simulink model "ADCS_sim"  (R2021b)
settings: Solver=VariableStepAuto  StartTime=0.0  StopTime=tf  RelTol=1e-3
values from neighbouring files (symbols this model uses):
  q_i = flip(quat)    [Jeri_Attitude_Prop.m]    (also in Nova_Attitude_Prop2.m = flip(q_i))
  w_i = [P;Q;R]    [Jeri_Attitude_Prop.m]    (also in Nova_Attitude_Prop2.m = [p;q;r])
undefined symbols (not defined in the file or in its folder): Params, qc, wc
libraries: sharedutil x1
settings Model: Creator=orena  LastModifiedBy=Tom
settings SolverCC: AlgebraicLoopSolver=TrustRegion
settings DebuggingCC: SFMachineParentedDataDiag=warning

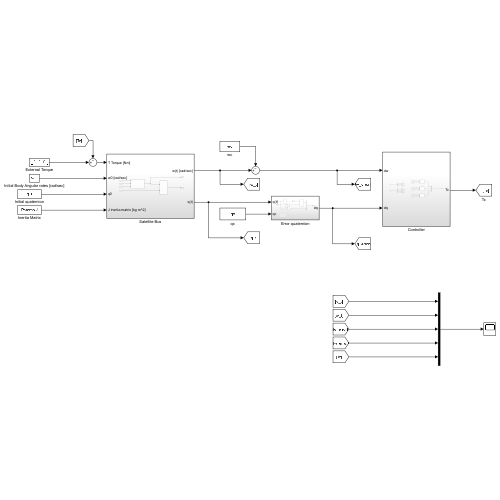
[thumbnail: Simulink's stored preview of the top-level diagram]
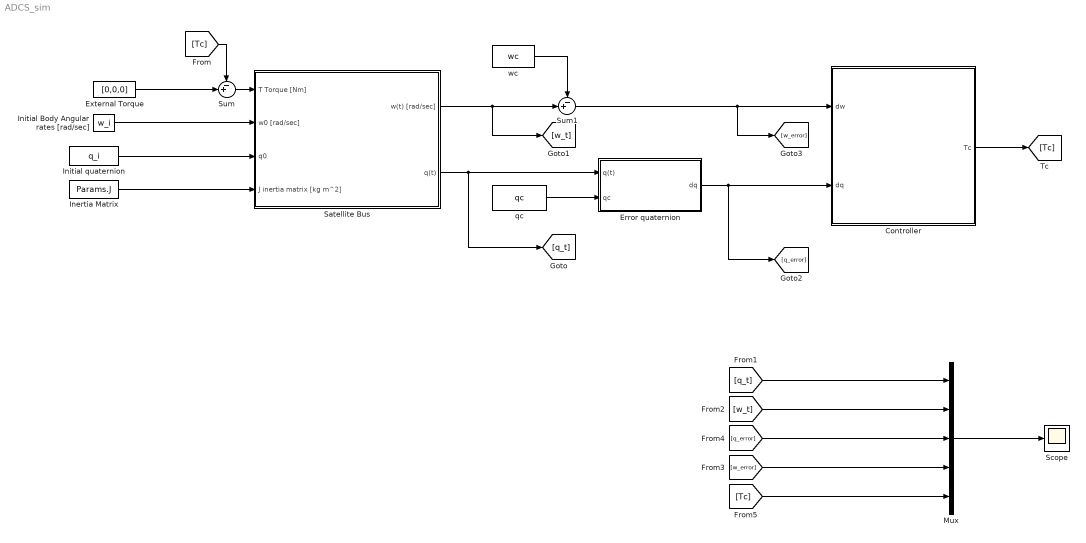
== system ADCS_sim ==
  Controller : Subsystem
  Error quaternion : Subsystem
  External Torque : Constant  Value=[0,0,0]
  Inertia Matrix : Constant  Value=Params.J
  Initial Body Angular rates [rad/sec] : Constant  Value=w_i
  Initial quaternion : Constant  Value=q_i
  Mux : Mux  Inputs=5
  Satellite Bus : Subsystem
  Scope : Scope
  Sum : Sum  Inputs=-+|
  Sum1 : Sum  Inputs=-+|
  qc : Constant  Value=qc
  wc : Constant  Value=wc
  wires:
  External Torque/1 -> Sum/2
  Controller/1(Tc) -> [Tc]
  [Tc] -> Sum/1
  wc/1 -> Sum1/1
  Sum/1 -> Satellite Bus/1(T Torque [Nm])
  Initial Body Angular rates [rad/sec]/1 -> Satellite Bus/2(w0 [rad/sec])
  Inertia Matrix/1 -> Satellite Bus/4(J inertia matrix [kg m^2])
  qc/1 -> Error quaternion/2(qc)
  Satellite Bus/2(q(t)) -> [q_t], Error quaternion/1(q(t))
  Error quaternion/1(dq) -> Controller/2(dq), [q_error]
  Satellite Bus/1(w(t) [rad/sec]) -> [w_t], Sum1/2
  Sum1/1 -> [w_error], Controller/1(dw)
  Initial quaternion/1 -> Satellite Bus/3(q0)
  [Tc] -> Mux/5
  [q_t] -> Mux/1
  [w_t] -> Mux/2
  [q_error] -> Mux/3
  [w_error] -> Mux/4
  Mux/1 -> Scope/1

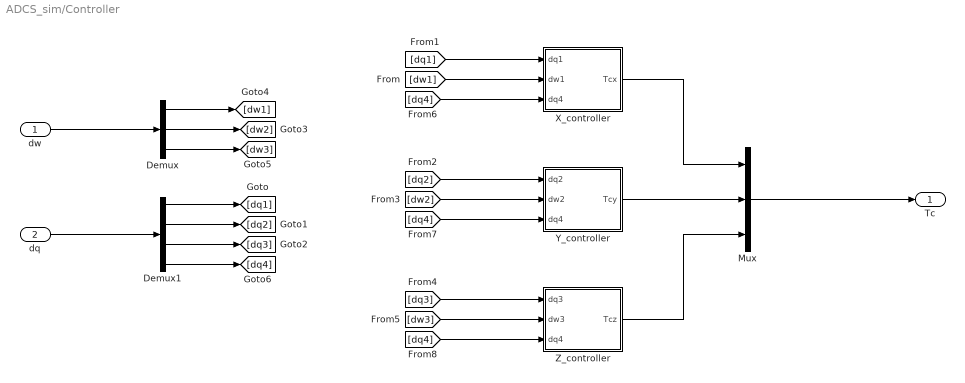
== system ADCS_sim/Controller ==
  dw : Inport
  dq : Inport  Port=2
  Demux : Demux  Outputs=3
  Demux1 : Demux
  Mux : Mux  Inputs=3
  X_controller : Subsystem
  Y_controller : Subsystem
  Z_controller : Subsystem
  Tc : Outport
  wires:
  Demux/1 -> [dw1]
  [dw2] -> Y_controller/2(dw2)
  [dq1] -> X_controller/1(dq1)
  [dq3] -> Z_controller/1(dq3)
  Demux/2 -> [dw2]
  Demux/3 -> [dw3]
  [dw3] -> Z_controller/2(dw3)
  Demux1/3 -> [dq3]
  Demux1/1 -> [dq1]
  Demux1/2 -> [dq2]
  [dq2] -> Y_controller/1(dq2)
  dw/1 -> Demux/1
  [dw1] -> X_controller/2(dw1)
  Y_controller/1(Tcy) -> Mux/2
  X_controller/1(Tcx) -> Mux/1
  Z_controller/1(Tcz) -> Mux/3
  Mux/1 -> Tc/1
  dq/1 -> Demux1/1
  Demux1/4 -> [dq4]
  [dq4] -> X_controller/3(dq4)
  [dq4] -> Y_controller/3(dq4)
  [dq4] -> Z_controller/3(dq4)

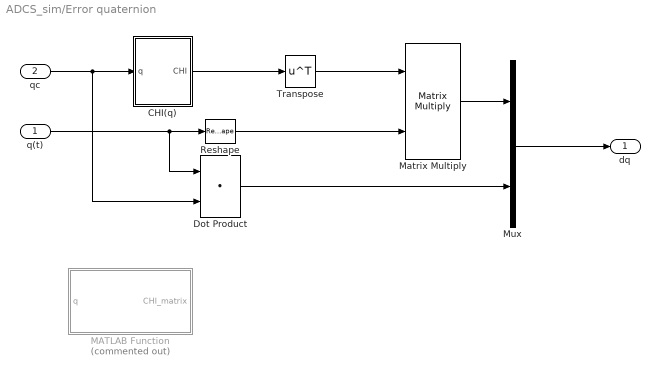
== system ADCS_sim/Error quaternion ==
  q(t) : Inport
  qc : Inport  Port=2
  CHI(q) : Subsystem
  Dot Product : DotProduct  InputSameDT=on  OutDataTypeStr=Inherit: Inherit via internal rule
  MATLAB Function : MATLAB Function  Commented=on  TreatAsAtomicUnit=on
  Matrix Multiply : Product  Multiplication=Matrix(*)
  Mux : Mux  Inputs=2
  Reshape : Reshape  OutputDimensionality=Column vector (2-D)
  Transpose : Math  Operator=transpose  SaturateOnIntegerOverflow=on
  dq : Outport
  wires:
  q(t)/1 -> Dot Product/1, Reshape/1
  Reshape/1 -> Matrix Multiply/2
  CHI(q)/1(CHI) -> Transpose/1
  qc/1 -> Dot Product/2, CHI(q)/1(q)
  Transpose/1 -> Matrix Multiply/1
  Matrix Multiply/1 -> Mux/1
  Mux/1 -> dq/1
  Dot Product/1 -> Mux/2

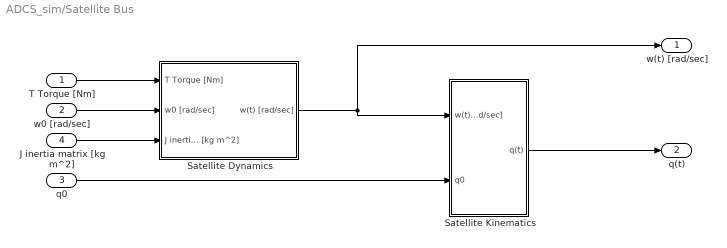
== system ADCS_sim/Satellite Bus ==
  T Torque [Nm] : Inport
  w0 [rad/sec] : Inport  Port=2
  q0 : Inport  Port=3
  J inertia matrix [kg m^2] : Inport  Port=4
  Satellite Dynamics : Subsystem
  Satellite Kinematics : Subsystem
  w(t) [rad/sec] : Outport
  q(t) : Outport  Port=2
  wires:
  q0/1 -> Satellite Kinematics/2(q0)
  Satellite Kinematics/1(q(t)) -> q(t)/1
  J inertia matrix [kg m^2]/1 -> Satellite Dynamics/3(J inertia matrix [kg m^2])
  w0 [rad/sec]/1 -> Satellite Dynamics/2(w0 [rad/sec])
  Satellite Dynamics/1(w(t) [rad/sec]) -> Satellite Kinematics/1(w(t) [rad/sec]), w(t) [rad/sec]/1
  T Torque [Nm]/1 -> Satellite Dynamics/1(T Torque [Nm])

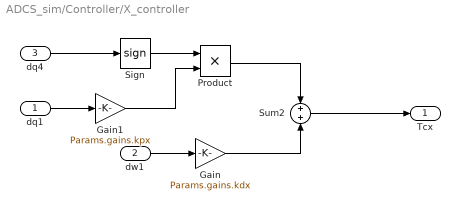
== system ADCS_sim/Controller/X_controller ==
  dq1 : Inport
  dw1 : Inport  Port=2
  dq4 : Inport  Port=3
  Gain : Gain  Gain=Params.gains.kdx
  Gain1 : Gain  Gain=Params.gains.kpx
  Product : Product
  Sign : Signum
  Sum2 : Sum  Inputs=+|+
  Tcx : Outport
  wires:
  Sum2/1 -> Tcx/1
  dq1/1 -> Gain1/1
  dw1/1 -> Gain/1
  Gain/1 -> Sum2/2
  dq4/1 -> Sign/1
  Sign/1 -> Product/1
  Gain1/1 -> Product/2
  Product/1 -> Sum2/1

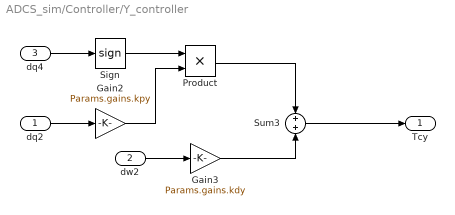
== system ADCS_sim/Controller/Y_controller ==
  dq2 : Inport
  dw2 : Inport  Port=2
  dq4 : Inport  Port=3
  Gain2 : Gain  Gain=Params.gains.kpy
  Gain3 : Gain  Gain=Params.gains.kdy
  Product : Product
  Sign : Signum
  Sum3 : Sum  Inputs=+|+
  Tcy : Outport
  wires:
  dq2/1 -> Gain2/1
  Gain3/1 -> Sum3/2
  Sum3/1 -> Tcy/1
  dw2/1 -> Gain3/1
  dq4/1 -> Sign/1
  Sign/1 -> Product/1
  Gain2/1 -> Product/2
  Product/1 -> Sum3/1

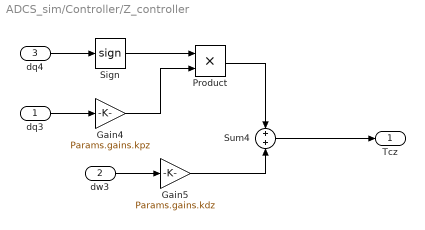
== system ADCS_sim/Controller/Z_controller ==
  dq3 : Inport
  dw3 : Inport  Port=2
  dq4 : Inport  Port=3
  Gain4 : Gain  Gain=Params.gains.kpz
  Gain5 : Gain  Gain=Params.gains.kdz
  Product : Product
  Sign : Signum
  Sum4 : Sum  Inputs=+|+
  Tcz : Outport
  wires:
  Sum4/1 -> Tcz/1
  dw3/1 -> Gain5/1
  Gain5/1 -> Sum4/2
  dq3/1 -> Gain4/1
  dq4/1 -> Sign/1
  Sign/1 -> Product/1
  Gain4/1 -> Product/2
  Product/1 -> Sum4/1

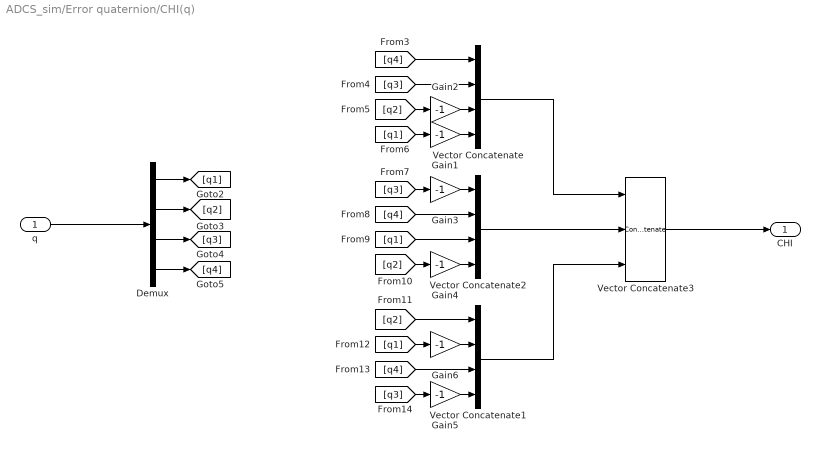
== system ADCS_sim/Error quaternion/CHI(q) ==
  q : Inport
  Demux : Demux
  Gain{1..6} (6 alike) : Gain  Gain=-1
  Vector Concatenate : Concatenate  NumInputs=4
  Vector Concatenate1 : Concatenate  NumInputs=4
  Vector Concatenate2 : Concatenate  NumInputs=4
  Vector Concatenate3 : Concatenate  NumInputs=3  Mode=Multidimensional array  ConcatenateDimension=2
  CHI : Outport
  wires:
  [q1] -> Vector Concatenate2/3
  [q3] -> Gain5/1
  Vector Concatenate3/1 -> CHI/1
  Vector Concatenate/1 -> Vector Concatenate3/1
  Vector Concatenate2/1 -> Vector Concatenate3/2
  q/1 -> Demux/1
  [q3] -> Gain3/1
  Gain3/1 -> Vector Concatenate2/1
  [q3] -> Vector Concatenate/2
  [q4] -> Vector Concatenate1/3
  [q1] -> Gain1/1
  Demux/2 -> [q2]
  Gain1/1 -> Vector Concatenate/4
  Demux/3 -> [q3]
  [q4] -> Vector Concatenate/1
  [q4] -> Vector Concatenate2/2
  Gain4/1 -> Vector Concatenate2/4
  [q2] -> Vector Concatenate1/1
  Demux/1 -> [q1]
  [q1] -> Gain6/1
  Gain6/1 -> Vector Concatenate1/2
  [q2] -> Gain2/1
  [q2] -> Gain4/1
  Gain2/1 -> Vector Concatenate/3
  Vector Concatenate1/1 -> Vector Concatenate3/3
  Demux/4 -> [q4]
  Gain5/1 -> Vector Concatenate1/4

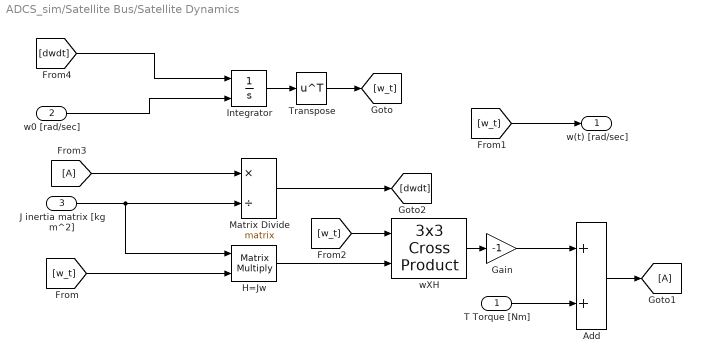
== system ADCS_sim/Satellite Bus/Satellite Dynamics ==
  T Torque [Nm] : Inport
  w0 [rad/sec] : Inport  Port=2
  J inertia matrix [kg m^2] : Inport  Port=3
  Add : Sum
  Gain : Gain  Gain=-1
  H=Jw : Product  Multiplication=Matrix(*)
  Integrator : Integrator  InitialConditionSource=external
  Matrix Divide : Product  Inputs=*/  Multiplication=Matrix(*)
  Transpose : Math  Operator=transpose  SaturateOnIntegerOverflow=on
  wXH : sharedutil/3x3 Cross Product  aMode=aMode
      settings: SourceProductBaseCode=AE,PW,DR,MT,UV,VE
  w(t) [rad/sec] : Outport
  wires:
  T Torque [Nm]/1 -> Add/2
  w0 [rad/sec]/1 -> Integrator/2
  Gain/1 -> Add/1
  [w_t] -> w(t) [rad/sec]/1
  Add/1 -> [A]
  J inertia matrix [kg m^2]/1 -> Matrix Divide/2, H=Jw/1
  H=Jw/1 -> wXH/2
  [dwdt] -> Integrator/1
  wXH/1 -> Gain/1
  [w_t] -> wXH/1
  [A] -> Matrix Divide/1
  Matrix Divide/1 -> [dwdt]
  [w_t] -> H=Jw/2
  Integrator/1 -> Transpose/1
  Transpose/1 -> [w_t]

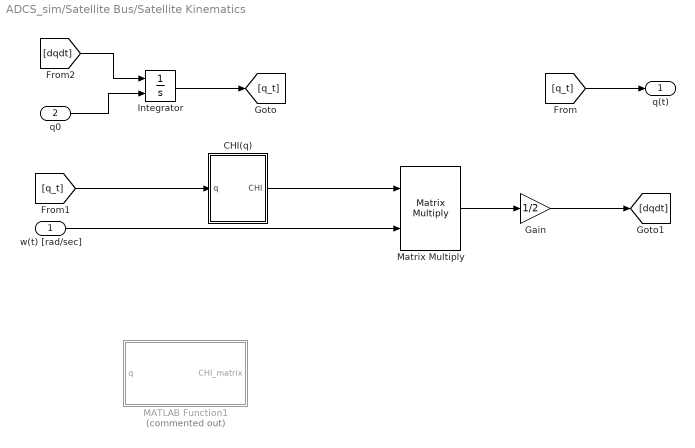
== system ADCS_sim/Satellite Bus/Satellite Kinematics ==
  w(t) [rad/sec] : Inport
  q0 : Inport  Port=2
  CHI(q) : Subsystem
  Gain : Gain  Gain=1/2
  Integrator : Integrator  InitialConditionSource=external
  MATLAB Function1 : MATLAB Function  Commented=on  TreatAsAtomicUnit=on
  Matrix Multiply : Product  Multiplication=Matrix(*)
  q(t) : Outport
  wires:
  [dqdt] -> Integrator/1
  [q_t] -> q(t)/1
  Gain/1 -> [dqdt]
  Integrator/1 -> [q_t]
  Matrix Multiply/1 -> Gain/1
  q0/1 -> Integrator/2
  w(t) [rad/sec]/1 -> Matrix Multiply/2
  CHI(q)/1(CHI) -> Matrix Multiply/1
  [q_t] -> CHI(q)/1(q)

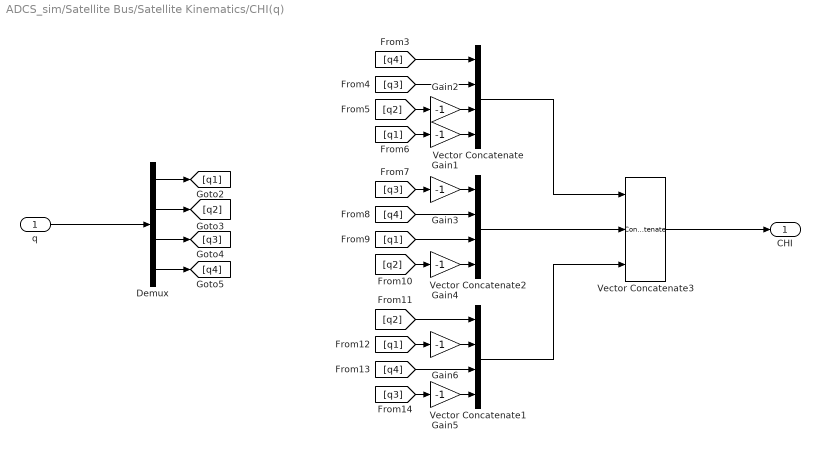
== system ADCS_sim/Satellite Bus/Satellite Kinematics/CHI(q) ==
  q : Inport
  Demux : Demux
  Gain{1..6} (6 alike) : Gain  Gain=-1
  Vector Concatenate : Concatenate  NumInputs=4
  Vector Concatenate1 : Concatenate  NumInputs=4
  Vector Concatenate2 : Concatenate  NumInputs=4
  Vector Concatenate3 : Concatenate  NumInputs=3  Mode=Multidimensional array  ConcatenateDimension=2
  CHI : Outport
  wires:
  [q1] -> Vector Concatenate2/3
  [q3] -> Gain5/1
  Vector Concatenate3/1 -> CHI/1
  Vector Concatenate/1 -> Vector Concatenate3/1
  Vector Concatenate2/1 -> Vector Concatenate3/2
  q/1 -> Demux/1
  [q3] -> Gain3/1
  Gain3/1 -> Vector Concatenate2/1
  [q3] -> Vector Concatenate/2
  [q4] -> Vector Concatenate1/3
  [q1] -> Gain1/1
  Demux/2 -> [q2]
  Gain1/1 -> Vector Concatenate/4
  Demux/3 -> [q3]
  [q4] -> Vector Concatenate/1
  [q4] -> Vector Concatenate2/2
  Gain4/1 -> Vector Concatenate2/4
  [q2] -> Vector Concatenate1/1
  Demux/1 -> [q1]
  [q1] -> Gain6/1
  Gain6/1 -> Vector Concatenate1/2
  [q2] -> Gain2/1
  [q2] -> Gain4/1
  Gain2/1 -> Vector Concatenate/3
  Vector Concatenate1/1 -> Vector Concatenate3/3
  Demux/4 -> [q4]
  Gain5/1 -> Vector Concatenate1/4

== matlab function ADCS_sim/Satellite Bus/Satellite Kinematics/MATLAB Function1 ==
  data: q input; CHI_matrix output
function CHI_matrix = CHI(q)

CHI_matrix = [q(4),-q(3),q(2);...
              q(3),q(4),-q(1);...
              -q(2),q(1),q(4);...
             -q(1),-q(2),-q(3)];

== matlab function ADCS_sim/Error quaternion/MATLAB Function ==
  data: q input; CHI_matrix output
function CHI_matrix = CHI(q)

CHI_matrix = [q(4),-q(3),q(2);...
              q(3),q(4),-q(1);...
              -q(2),q(1),q(4);...
             -q(1),-q(2),-q(3)];
